simulink model "notifbatreirobot"  (R2016a)
settings: Solver=VariableStepAuto  StartTime=0.0  StopTime=inf  RelTol=1e-3
settings Model: Creator=Ms  LastModifiedBy=Ms

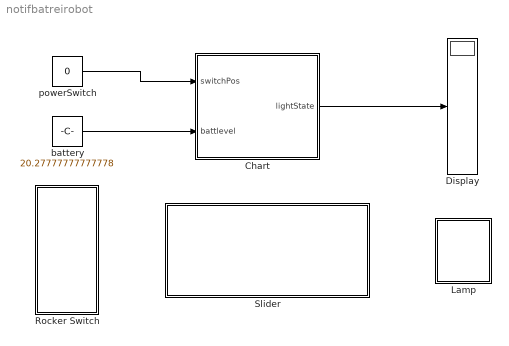
== system notifbatreirobot ==
  Chart : Stateflow chart  TreatAsAtomicUnit=on
  Display : Display
  Lamp : Subsystem  DialogController=hmiCreateDDGDialog  IsWebBlock=on  mask(MWDashboardBlock){webBlockId=6b6217f7-8ea5-483a-a856-5edce2452137, webBlockType=lamp, ShowInLibBrowser=on, ShowInitialText=on, HMISrcModelName=notifbatreirobot}
      mask prompts: webBlockType "WebBlock Type"; HMISrcModelName "Source Model"
      mask Help: helpview([docroot '/mapfiles/simulink.map'], 'hmi_lamp')
      mask Display:
      | if strcmp(get_param(bdroot(gcb),'BlockDiagramType'), 'library')
      |     image([(matlabroot) '/toolbox/simulink/hmi/icons/Lamp.png']);
      | end
  Rocker Switch : Subsystem  DialogController=hmiCreateDDGDialog  IsWebBlock=on  mask(MWDashboardBlock){webBlockId=6805bf21-afa8-494a-871a-a5a7f54a263f, webBlockType=rockerswitch, ShowInLibBrowser=on, ShowInitialText=on, HMISrcModelName=notifbatreirobot}
      mask prompts: webBlockId "WebBlock Id"; webBlockType "WebBlock Type"; HMISrcModelName "Source Model"
      mask Help: helpview([docroot '/mapfiles/simulink.map'], 'hmi_rocker_switch')
      mask Display:
      | if strcmp(get_param(bdroot(gcb),'BlockDiagramType'), 'library')
      |     image([(matlabroot) '/toolbox/simulink/hmi/icons/RockerSwitch.png']);
      | end
  Slider : Subsystem  DialogController=hmiCreateDDGDialog  IsWebBlock=on  mask(MWDashboardBlock){webBlockId=6465138f-51e6-4dc9-adb4-8067bff19bad, webBlockType=slider, ShowInLibBrowser=on, ShowInitialText=on, HMISrcModelName=notifbatreirobot}
      mask prompts: webBlockId "WebBlock Id"; webBlockType "WebBlock Type"; HMISrcModelName "Source Model"
      mask Help: helpview([docroot '/mapfiles/simulink.map'], 'hmi_slider')
      mask Display:
      | if strcmp(get_param(bdroot(gcb),'BlockDiagramType'), 'library')
      |     image([(matlabroot) '/toolbox/simulink/hmi/icons/Slider.png']);
      | end
  battery : Constant  Value=20.27777777777778
  powerSwitch : Constant  Value=0
  wires:
  powerSwitch/1 -> Chart/1(switchPos)
  battery/1 -> Chart/2(battlevel)
  Chart/1(lightState) -> Display/1

== system notifbatreirobot/Lamp ==

== system notifbatreirobot/Rocker Switch ==

== system notifbatreirobot/Slider ==

== stateflow chart notifbatreirobot/Chart ==
  state OFF1
    entry:
    lightState=0;
  state ON
    entry:
    lightState=1;
  state LOW_BATT
    entry:
    lightState=2;
  (default) -> OFF1
  OFF1 -> ON : [switchPos==1]
  ON -> OFF1 [order 1] : [switchPos==0]
  (junction 11) -> OFF1
  ON -> (junction 13) [order 2] : [battlevel<10]
  LOW_BATT -> (junction 11) : after(3,sec)
  (junction 13) -> LOW_BATT
  data: switchPos input; battlevel input; lightState output
